simulink library "Lib_Dyn_BiasedNRSolver_EMTAT"  (R2020b)
settings: Solver=ode45  StartTime=0.0  StopTime=10.0  RelTol=1e-3  EnableMultiTasking=on
undefined symbols (not defined in the file): SJac_Per_I
libraries: Lib_NM_NewtonRaphsonSolver_EMTAT x1
settings Model: Creator=jlkratz  LastModifiedBy=mebell
settings DataIOCC: LimitDataPoints=on  SaveFormat=Array  ReturnWorkspaceOutputs=off
settings OptimizationCC: LifeSpan=inf
settings DebuggingCC: SFUnexpectedBacktrackingDiag=warning  SFNoUnconditionalDefaultTransitionDiag=warning  SFExecutionAtInitializationDiag=none  ArithmeticOperatorsInVariantConditions=warning
settings HardwareCC: ProdBitPerPointer=32  ProdBitPerSizeT=32  ProdBitPerPtrDiffT=32  ProdLargestAtomicFloat=None  ProdIntDivRoundTo=Undefined  ProdEndianess=Unspecified  ProdWordSize=32  ProdHWDeviceType=32-bit Generic
settings ModelReferenceCC: PropagateSignalLabelsOutOfModel=off
settings SFSimCC: SimUseLocalCustomCode=off  CustomCodeUndefinedFunction=UseInterfaceOnly
settings RTWCC: RTWUseLocalCustomCode=off
settings CodeAppCC: StateflowObjectComments=on
settings GRTTargetCC: TargetLangStandard=C89/C90 (ANSI)
settings ConfigComp: CovMetricSettings=dw  CovSaveCumulativeToWorkspaceVar=on  CovSaveSingleToWorkspaceVar=on  CovExternalEMLEnable=off

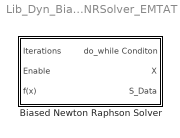
== system Lib_Dyn_BiasedNRSolver_EMTAT ==
  Biased Newton Raphson Solver : Subsystem  mask(Newton Raphson Solver){SJac_Per_M=[0.01 0.01 0.01; -0.01 -0.01 -0.01], SNR_IC_M=[1.5; 0.8; 0.7], Shift_M=5, SNR_DX_M=5, SNR_Mx_M=100000000, SNR_Mn_M=-100000000, SJacobianAttempts_M=1, Cond_Limits_M=0.01}
      mask prompts: SJac_Per_M "SJac_Per_M - Jacobian Perturbation size (frac) (nxm)"; SNR_IC_M "SNR_IC_M - Newton Raphson Initial Conditions (mx1)"; Shift_M "Shift_M - Bias to shift the solution to avoid convergence issues"; SNR_DX_M "SNR_DX_M - Newton Raphson step size limiter (%) (1x1)"; SNR_Mx_M "SNR_Mx_M - Newton Raphson max limit (1x1 or mx1)"; SNR_Mn_M "SNR_Mn_M - Newton Raphson min limit (1x1 or mx1)"; SJacobianAttempts_M "SJacobianAttempts_M - Newton Raphson attempts before the Jacobian recalculation (1x1)"; Cond_Limits_M "Cond_Limits_M - Iteration Conditions Limits (mx1 or 1x1)"
      mask help:
      | The Iterative Newton Raphson Solver with Jacobian Calculator block will
      | supply the inputs to iteratively drive the outputs of a system to zero.
      |
      | This will be performed in three steps.
      | 1) Jabobian calculator sends Perturbations to the plant then calculates the plant
      | Jacboian based on the system response
      | 2) The Newton Raphson will use the inverse of the Jacobian to iteratively step the
      | system toward solution.
      | 3) Once the solution has satisfied the conditions the Newton Raphson is shut off.
      |
      | This module is designed for dynamic systems and should be paired with
      | a "do... while" block in Simulink. The "do...while" block and this module
      | should both be located in the same subsystem as the plant that is to be solved for.
      mask init:
      | if isequal(size(SNR_Mx_M),size(SNR_IC_M))
      | elseif isequal(size(SNR_Mx_M),[1 1])
      | else
      |     disp('NR_Mx_Lim_M must be the same size as NR_IC_M or a constant')
      | end
      | 
      | if isequal(size(SNR_Mn_M),size(SNR_IC_M))
      | elseif isequal(size(SNR_Mn_M),[1 1])
      | else
      |     disp('NR_Mn_Lim_M must be the same size as NR_IC_M or a constant')
      | end
      | 
      | for i = 1:size(SJac_Per_M,1)
      |     SJac_Per_I(i,:) = SJac_Per_M(i,:).*(SNR_IC_M'./(SNR_IC_M' + Shift_M));
      | end
      mask Help: web(which('Solver_TMATS_INRSwJC.html'),'-helpbrowser')

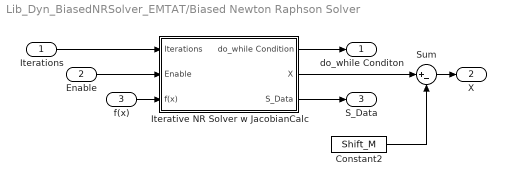
== system Lib_Dyn_BiasedNRSolver_EMTAT/Biased Newton Raphson Solver ==
  Iterations : Inport
  Enable : Inport  Port=2
  f(x) : Inport  Port=3
  Constant2 : Constant  Value=Shift_M
  Iterative NR Solver w JacobianCalc : Subsystem  mask(T-MATS: Iterative NR Solver w Jacobian Calc Library Block){SJac_Per_M=SJac_Per_I, SNR_IC_M=SNR_IC_M + Shift_M, SNR_DX_M=SNR_DX_M, SNR_Mx_M=SNR_Mx_M, SNR_Mn_M=SNR_Mn_M, SJacobianAttempts_M=SJacobianAttempts_M, Cond_Limits_M=Cond_Limits_M}
      mask prompts: SJac_Per_M "SJac_Per_M - Jacobian Perturbation size (frac) (nxm)"; SNR_IC_M "SNR_IC_M - Newton Raphson Initial Conditions (mx1)"; SNR_DX_M "SNR_DX_M - Newton Raphson step size limiter (%) (1x1)"; SNR_Mx_M "SNR_Mx_M - Newton Raphson max limit (1x1 or mx1)"; SNR_Mn_M "SNR_Mn_M - Newton Raphson min limit (1x1 or mx1)"; SJacobianAttempts_M "SJacobianAttempts_M - Newton Raphson attempts before the Jacobian recalculation (1x1)"; Cond_Limits_M "Cond_Limits_M - Iteration Conditions Limits (mx1 or 1x1)"
      mask help:
      | The Iterative Newton Raphson Solver with Jacobian Calculator block will
      | supply the inputs to iteratively drive the outputs of a system to zero.
      |
      | This will be performed in three steps.
      | 1) Jabobian calculator sends Perturbations to the plant then calculates the plant
      | Jacboian based on the system response
      | 2) The Newton Raphson will use the inverse of the Jacobian to iteratively step the
      | system toward solution.
      | 3) Once the solution has satisfied the conditions the Newton Raphson is shut off.
      |
      | This module is designed for dynamic systems and should be paired with
      | a "do... while" block in Simulink. The "do...while" block and this module
      | should both be located in the same subsystem as the plant that is to be solved for.
      mask init:
      | if isequal(size(SNR_Mx_M),size(SNR_IC_M))
      | elseif isequal(size(SNR_Mx_M),[1 1])
      | else
      |     disp('NR_Mx_Lim_M must be the same size as NR_IC_M or a constant')
      | end
      | 
      | if isequal(size(SNR_Mn_M),size(SNR_IC_M))
      | elseif isequal(size(SNR_Mn_M),[1 1])
      | else
      |     disp('NR_Mn_Lim_M must be the same size as NR_IC_M or a constant')
      | end
      mask Help: web(which('Solver_TMATS_INRSwJC.html'),'-helpbrowser')
  Sum : Sum  Inputs=|+-
  do_while Conditon : Outport
  X : Outport  Port=2
  S_Data : Outport  Port=3
  wires:
  Sum/1 -> X/1
  Iterative NR Solver w JacobianCalc/1(do_while Condition) -> do_while Conditon/1
  Iterative NR Solver w JacobianCalc/3(S_Data) -> S_Data/1
  Enable/1 -> Iterative NR Solver w JacobianCalc/2(Enable)
  Iterations/1 -> Iterative NR Solver w JacobianCalc/1(Iterations)
  f(x)/1 -> Iterative NR Solver w JacobianCalc/3(f(x))
  Iterative NR Solver w JacobianCalc/2(X) -> Sum/1
  Constant2/1 -> Sum/2

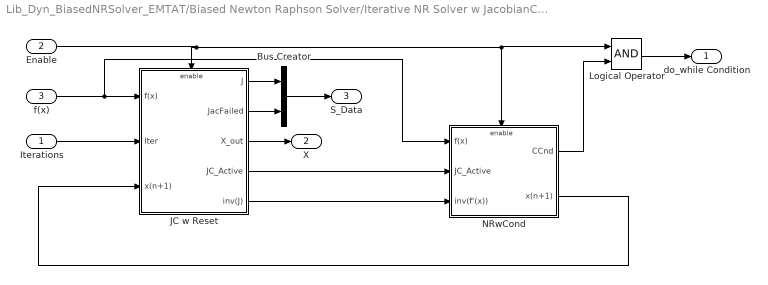
== system Lib_Dyn_BiasedNRSolver_EMTAT/Biased Newton Raphson Solver/Iterative NR Solver w JacobianCalc ==
  Iterations : Inport  PortDimensions=1
  Enable : Inport  Port=2  PortDimensions=1
  f(x) : Inport  Port=3  PortDimensions=length(SNR_IC_M)
  Bus Creator : BusCreator  Inputs=2
  JC w Reset : Subsystem
  Logical Operator : Logic  AllPortsSameDT=off  OutDataTypeStr=boolean
  NRwCond : Subsystem
  do_while Condition : Outport  PortDimensions=1
  X : Outport  Port=2  PortDimensions=length(SNR_IC_M)
  S_Data : Outport  Port=3
  wires:
  JC w Reset/2(JacFailed) -> Bus Creator/2
  Bus Creator/1 -> S_Data/1
  Logical Operator/1 -> do_while Condition/1
  Enable/1 -> Logical Operator/1, NRwCond/Enable, JC w Reset/Enable
  JC w Reset/5(inv(J)) -> NRwCond/3(inv(f'(x)))
  JC w Reset/4(JC_Active) -> NRwCond/2(JC_Active)
  JC w Reset/3(X_out) -> X/1
  JC w Reset/1(J) -> Bus Creator/1
  NRwCond/2(x(n+1)) -> JC w Reset/3(x(n+1))
  Iterations/1 -> JC w Reset/2(Iter)
  NRwCond/1(CCnd) -> Logical Operator/2
  f(x)/1 -> NRwCond/1(f(x)), JC w Reset/1(f(x))

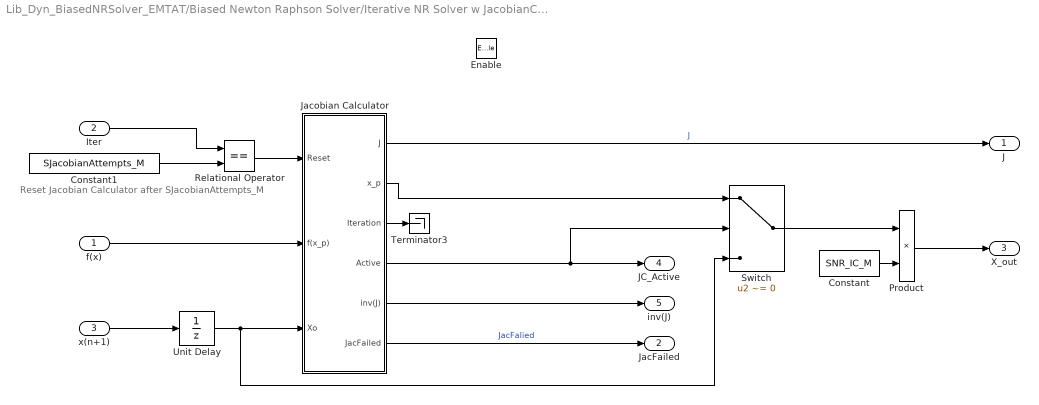
== system Lib_Dyn_BiasedNRSolver_EMTAT/Biased Newton Raphson Solver/Iterative NR Solver w JacobianCalc/JC w Reset ==
  note: Reset Jacobian Calculator after SJacobianAttempts_M
  f(x) : Inport  PortDimensions=length(SNR_IC_M)
  Iter : Inport  Port=2  PortDimensions=1
  x(n+1) : Inport  Port=3
  Enable : EnablePort
  Constant : Constant  Value=SNR_IC_M
  Constant1 : Constant  Value=SJacobianAttempts_M  OutDataTypeStr=uint32
  Jacobian Calculator : Subsystem  TreatAsAtomicUnit=on  mask(T-MATS: Jacobian Calculator Library Block){N_Per_M=SJac_Per_M}
      mask prompts: N_Per_M "N_Per_M - Perturbations (nxm)"
      mask help:
      | The Jacobian Calculator block calculates the Jabobian of the system by perturbing the system around an initial point and calculating the gradient for each perturbation. This module will run once on start up and then again only if the reset is pressed.
      | Below: n (rows) is the number of times each independent will be perturbed and m (columns) is the number of inputs.
      mask Help: web(which('NumMthd_TMATS_JC.html'),'-helpbrowser')
  Product : Product  RndMeth=Zero
  Relational Operator : RelationalOperator  Operator===  OutDataTypeStr=boolean  RndMeth=Nearest
  Switch : Switch  Criteria=u2 ~= 0  Threshold=1
  Terminator3 : Terminator
  Unit Delay : UnitDelay  InitialCondition=ones(length(SNR_IC_M),1)  SampleTime=-1  HasFrameUpgradeWarning=on
  J : Outport  PortDimensions=[length(SNR_IC_M),length(SNR_IC_M)]
  JacFailed : Outport  Port=2  PortDimensions=1
  X_out : Outport  Port=3  PortDimensions=length(SNR_IC_M)
  JC_Active : Outport  Port=4  PortDimensions=1
  inv(J) : Outport  Port=5  PortDimensions=[length(SNR_IC_M),length(SNR_IC_M)]
  wires:
  Jacobian Calculator/6(JacFailed) -> JacFailed/1  "JacFalied"
  Jacobian Calculator/3(Iteration) -> Terminator3/1
  Iter/1 -> Relational Operator/1
  Constant1/1 -> Relational Operator/2
  Jacobian Calculator/4(Active) -> JC_Active/1, Switch/2
  Switch/1 -> Product/1
  Jacobian Calculator/2(x_p) -> Switch/1
  Product/1 -> X_out/1
  Relational Operator/1 -> Jacobian Calculator/1(Reset)
  Constant/1 -> Product/2
  Jacobian Calculator/1(J) -> J/1  "J"
  x(n+1)/1 -> Unit Delay/1
  Unit Delay/1 -> Jacobian Calculator/3(Xo), Switch/3
  Jacobian Calculator/5(inv(J)) -> inv(J)/1
  f(x)/1 -> Jacobian Calculator/2(f(x_p))

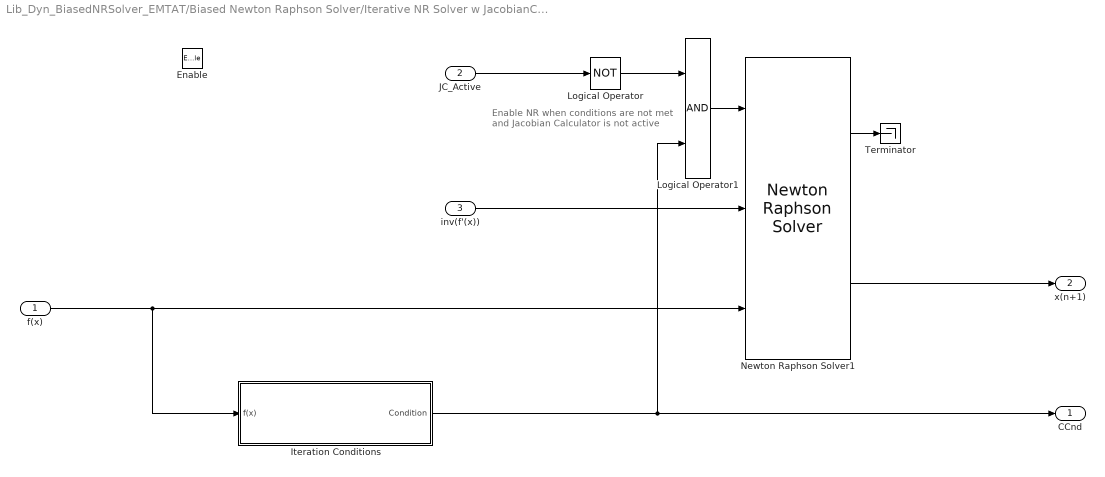
== system Lib_Dyn_BiasedNRSolver_EMTAT/Biased Newton Raphson Solver/Iterative NR Solver w JacobianCalc/NRwCond ==
  note: Enable NR when conditions are not met
      | and Jacobian Calculator is not active
  f(x) : Inport  PortDimensions=length(SNR_IC_M)
  JC_Active : Inport  Port=2  PortDimensions=1
  inv(f'(x)) : Inport  Port=3  PortDimensions=[length(SNR_IC_M),length(SNR_IC_M)]
  Enable : EnablePort
  Iteration Conditions : Subsystem
  Logical Operator : Logic  Operator=NOT  AllPortsSameDT=off  OutDataTypeStr=boolean
  Logical Operator1 : Logic  AllPortsSameDT=off  OutDataTypeStr=boolean
  Newton Raphson Solver1 : Lib_NM_NewtonRaphsonSolver_EMTAT/Newton Raphson Solver  NR_IC_M=SNR_IC_M./abs(SNR_IC_M)  NR_dx_Lim_M=SNR_DX_M  NR_Mx_Lim_M=SNR_Mx_M./abs(SNR_IC_M)  NR_Mn_Lim_M=SNR_Mn_M./abs(SNR_IC_M)  BlkNm_M=double(gcb)
  Terminator : Terminator
  CCnd : Outport  PortDimensions=1
  x(n+1) : Outport  Port=2  PortDimensions=length(SNR_IC_M)
  wires:
  Iteration Conditions/1(Condition) -> CCnd/1, Logical Operator1/2
  Logical Operator/1 -> Logical Operator1/1
  Logical Operator1/1 -> Newton Raphson Solver1/1
  inv(f'(x))/1 -> Newton Raphson Solver1/2
  Newton Raphson Solver1/1 -> Terminator/1
  Newton Raphson Solver1/2 -> x(n+1)/1
  JC_Active/1 -> Logical Operator/1
  f(x)/1 -> Newton Raphson Solver1/3, Iteration Conditions/1(f(x))

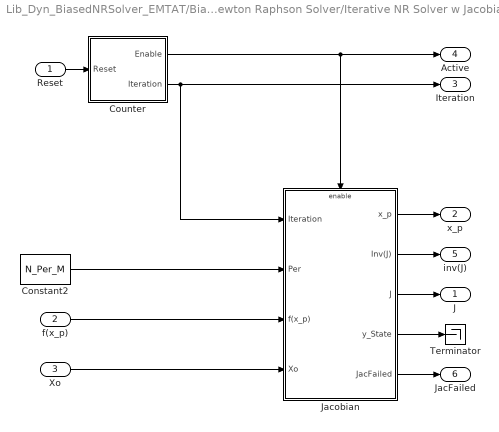
== system Lib_Dyn_BiasedNRSolver_EMTAT/Biased Newton Raphson Solver/Iterative NR Solver w JacobianCalc/JC w Reset/Jacobian Calculator ==
  Reset : Inport  PortDimensions=1
  f(x_p) : Inport  Port=2  PortDimensions=size(N_Per_M,2)
  Xo : Inport  Port=3  PortDimensions=size(N_Per_M,2)
  Constant2 : Constant  Value=N_Per_M
  Counter : Subsystem  mask{N_Ind_M=prod(size(N_Per_M))}
      mask prompts: N_Ind_M "number of independents, N_Ind_M"
  Jacobian : Subsystem
  Terminator : Terminator
  J : Outport  PortDimensions=[size(N_Per_M,2), size(N_Per_M,2)]
  x_p : Outport  Port=2  PortDimensions=size(N_Per_M,2)
  Iteration : Outport  Port=3  PortDimensions=1
  Active : Outport  Port=4  PortDimensions=1
  inv(J) : Outport  Port=5  PortDimensions=[size(N_Per_M,2), size(N_Per_M,2)]
  JacFailed : Outport  Port=6  PortDimensions=1
  wires:
  Jacobian/5(JacFailed) -> JacFailed/1
  Jacobian/4(y_State) -> Terminator/1
  Jacobian/3(J) -> J/1
  Jacobian/2(Inv(J)) -> inv(J)/1
  Counter/2(Iteration) -> Jacobian/1(Iteration), Iteration/1
  Xo/1 -> Jacobian/4(Xo)
  Counter/1(Enable) -> Jacobian/Enable, Active/1
  Reset/1 -> Counter/1(Reset)
  Jacobian/1(x_p) -> x_p/1
  Constant2/1 -> Jacobian/2(Per)
  f(x_p)/1 -> Jacobian/3(f(x_p))

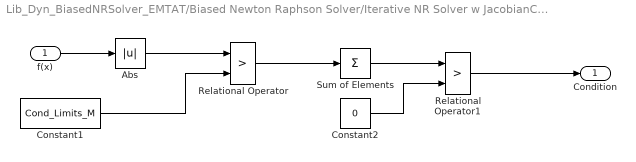
== system Lib_Dyn_BiasedNRSolver_EMTAT/Biased Newton Raphson Solver/Iterative NR Solver w JacobianCalc/NRwCond/Iteration Conditions ==
  f(x) : Inport
  Abs : Abs
  Constant1 : Constant  Value=Cond_Limits_M
  Constant2 : Constant  Value=0
  Relational Operator : RelationalOperator  Operator=>  OutDataTypeStr=boolean  RndMeth=Nearest
  Relational Operator1 : RelationalOperator  Operator=>  OutDataTypeStr=boolean  RndMeth=Nearest
  Sum of Elements : Sum  Inputs=+
  Condition : Outport
  wires:
  Abs/1 -> Relational Operator/1
  Constant1/1 -> Relational Operator/2
  f(x)/1 -> Abs/1
  Relational Operator/1 -> Sum of Elements/1
  Constant2/1 -> Relational Operator1/2
  Sum of Elements/1 -> Relational Operator1/1
  Relational Operator1/1 -> Condition/1

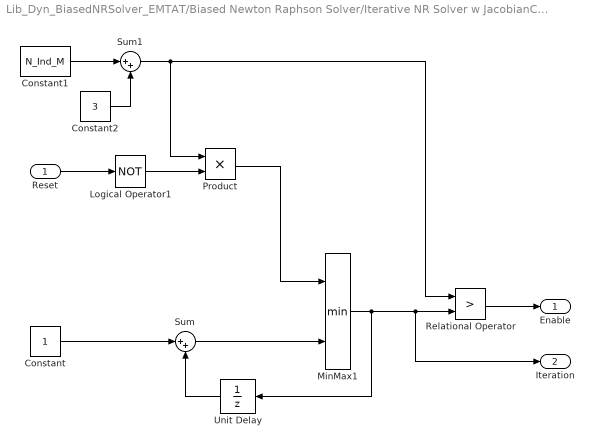
== system Lib_Dyn_BiasedNRSolver_EMTAT/Biased Newton Raphson Solver/Iterative NR Solver w JacobianCalc/JC w Reset/Jacobian Calculator/Counter ==
  Reset : Inport
  Constant : Constant
  Constant1 : Constant  Value=N_Ind_M
  Constant2 : Constant  Value=3
  Logical Operator1 : Logic  Operator=NOT  AllPortsSameDT=off  OutDataTypeStr=boolean
  MinMax1 : MinMax  Inputs=2
  Product : Product  RndMeth=Zero
  Relational Operator : RelationalOperator  Operator=>  OutDataTypeStr=boolean  RndMeth=Nearest
  Sum : Sum  Inputs=|++
  Sum1 : Sum  Inputs=|++
  Unit Delay : UnitDelay  SampleTime=-1  HasFrameUpgradeWarning=on
  Enable : Outport
  Iteration : Outport  Port=2
  wires:
  Constant1/1 -> Sum1/1
  Constant2/1 -> Sum1/2
  Sum1/1 -> Product/1, Relational Operator/1
  Reset/1 -> Logical Operator1/1
  Logical Operator1/1 -> Product/2
  Relational Operator/1 -> Enable/1
  MinMax1/1 -> Relational Operator/2, Iteration/1, Unit Delay/1
  Unit Delay/1 -> Sum/2
  Sum/1 -> MinMax1/2
  Product/1 -> MinMax1/1
  Constant/1 -> Sum/1

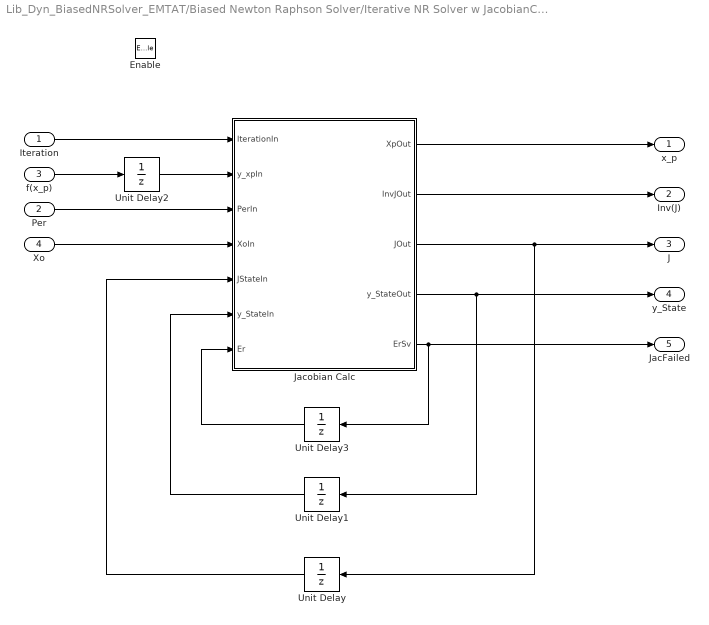
== system Lib_Dyn_BiasedNRSolver_EMTAT/Biased Newton Raphson Solver/Iterative NR Solver w JacobianCalc/JC w Reset/Jacobian Calculator/Jacobian ==
  Iteration : Inport
  Per : Inport  Port=2
  f(x_p) : Inport  Port=3
  Xo : Inport  Port=4
  Enable : EnablePort
  Jacobian Calc : MATLAB Function  TreatAsAtomicUnit=on
  Unit Delay : UnitDelay  InitialCondition=zeros(size(N_Per_M,2),size(N_Per_M,2))  SampleTime=-1  HasFrameUpgradeWarning=on
  Unit Delay1 : UnitDelay  InitialCondition=zeros(size(N_Per_M,2),prod(size(N_Per_M))+1)  SampleTime=-1  HasFrameUpgradeWarning=on
  Unit Delay2 : UnitDelay  InitialCondition=zeros(size(N_Per_M,2),1)  SampleTime=-1  HasFrameUpgradeWarning=on
  Unit Delay3 : UnitDelay  SampleTime=-1  HasFrameUpgradeWarning=on
  x_p : Outport
  Inv(J) : Outport  Port=2
  J : Outport  Port=3
  y_State : Outport  Port=4
  JacFailed : Outport  Port=5
  wires:
  Unit Delay3/1 -> Jacobian Calc/7(Er)
  Jacobian Calc/5(ErSv) -> JacFailed/1, Unit Delay3/1
  Unit Delay2/1 -> Jacobian Calc/2(y_xpIn)
  f(x_p)/1 -> Unit Delay2/1
  Unit Delay1/1 -> Jacobian Calc/6(y_StateIn)
  Jacobian Calc/4(y_StateOut) -> y_State/1, Unit Delay1/1
  Unit Delay/1 -> Jacobian Calc/5(JStateIn)
  Jacobian Calc/2(InvJOut) -> Inv(J)/1
  Jacobian Calc/3(JOut) -> J/1, Unit Delay/1
  Iteration/1 -> Jacobian Calc/1(IterationIn)
  Per/1 -> Jacobian Calc/3(PerIn)
  Xo/1 -> Jacobian Calc/4(XoIn)
  Jacobian Calc/1(XpOut) -> x_p/1

== matlab function Lib_Dyn_BiasedNRSolver_EMTAT/Biased Newton Raphson Solver/Iterative NR Solver w JacobianCalc/JC w Reset/Jacobian Calculator/Jacobian/Jacobian Calc ==
  data: IterationIn input; XpOut output; y_xpIn input; PerIn input; XoIn input; InvJOut output; JOut output; JStateIn input; y_StateIn input; y_StateOut output; Er input; ErSv output
function [XpOut, InvJOut, JOut, y_StateOut, ErSv] = fcn(IterationIn, y_xpIn, PerIn, XoIn, JStateIn, y_StateIn, Er)

% Set inital condiations
i = IterationIn;
XpOut = XoIn;
InvJOut = zeros(length(XoIn));
JOut = JStateIn;
y_StateOut = y_StateIn;
PerVec = reshape(PerIn',1,[]);
LenPV = length(PerVec);
LenXo = length(XoIn);
ErSv = Er;

% Begin taking data from f(x) at iteration a+1
a = 1;
% Begin determining Jacobian at iteration b+1
b = a+1;

% Set Xp Output
if i > a && i <= LenPV + a
    current_Xp = mod(i-a-1,LenXo)+1;
    XpOut(current_Xp) = XpOut(current_Xp) + PerVec(i - a);
end

% save state feedback
if LenXo == 1
    if i >= b;
        y_StateOut(i-a) = y_xpIn;
    end
else
    if i > a && i<= LenPV + a+1;
        y_StateOut(:,i - a) = y_xpIn;
    end
end

% Create Jacobian
if i == LenPV + b
    % Generate Jacobian matrices for each set, stacked.
    if LenXo == 1
        JMtx_extended = (y_StateOut(2:end)' - repmat(y_StateOut(1),1,LenPV))./PerVec;
    else
        JMtx_extended = (y_StateOut(:,2:end) - repmat(y_StateOut(:,1),1,LenPV))./repmat(PerVec,LenXo,1);
    end
    
    % Initialize sum matricies
    JMtrx_sum = zeros(LenXo);
    Nsum = zeros(LenXo);
    
    % determine how many perturbation sets there are, b/c MATLAB likes to
    % flip vectors when they enter MATLAB functions from Simulink for no reason.
    if min(size(PerIn)) == 1
     if LenXo == 1;
        PerNum = length(PerIn); 
     else 
        PerNum = 1;
     end
    else
        PerNum = size(PerIn,1);
    end
    
    for set = 1: PerNum
        % Break out Jacobian matrix for the current perturbation set
        JMtrx_cur = JMtx_extended(:, LenXo*(set-1)+1:LenXo*set);
        % Sum Jacobian matrices for each set
        JMtrx_sum = JMtrx_sum + JMtrx_cur(:,1:LenXo);
        % Sum number of acceptable values
        Nsum = Nsum + abs(sign(JMtrx_cur(:,1:LenXo)));
    end
    
    % Average Jacobian Matricies
    Javg = JMtrx_sum./max(Nsum,1);
    
    JOut = Javg;
    
    % Invert Jacobian
    if rank(JOut) == length(InvJOut)
        InvJOut = inv(JOut(:,:));
    elseif ErSv < 1
        disp('Jacobian can not be inverted.');
        ErSv = 1;
    end
end
